simulink model "cube_3d_simulation_model_fast_mpc"  (R2016b)
settings: Solver=VariableStepAuto  StartTime=0.0  StopTime=2  RelTol=1e-3  EnableMultiTasking=on
model workspace (MAT data in the model file):
  Sig = Simulink.Signal
  Sig.DataType = 'double'
  Sig.Dimensions = -1
  Sig.DimensionsMode = 'auto'
  Sig.Complexity = 'auto'
  Sig.SampleTime = -1
  Sig.SamplingMode = 'auto'
values from neighbouring files (symbols this model uses):
  cog_offs = zeros(3,1)    [Fast_MPC_3d_Linear_system.m]    (also in Run_FastMPC_Nonlinear_model.m = theta_offs*norm(cube.rcb)*e_cog_offs)
  phi0 = deg2rad(2)    [Fast_MPC_3d_Linear_system.m]    (also in Run_FastMPC_Nonlinear_model.m = deg2rad(1.5))
  phi00 = 0    [Fast_MPC_3d_Linear_system.m]    (also in Run_FastMPC_Nonlinear_model.m)
  psi0 = deg2rad(2)    [Fast_MPC_3d_Linear_system.m]    (also in Run_FastMPC_Nonlinear_model.m = deg2rad(-1.5))
  psi00 = pi/4    (= 0.785398163397)    [Fast_MPC_3d_Linear_system.m]    (also in Run_FastMPC_Nonlinear_model.m)
  theta0 = deg2rad(2)    [Fast_MPC_3d_Linear_system.m]    (also in MPC_Parameters_3D.m = atan(sqrt(2)); Run_FastMPC_Nonlinear_model.m = deg2rad(1.5))
  theta00 = atan(sqrt(2))    [Fast_MPC_3d_Linear_system.m]    (also in Run_FastMPC_Nonlinear_model.m)
  Ts = Ts.controller    [MPC_Parameters_3D.m]
undefined symbols (not defined in the file or in its folder): cube, motor, Q0, wheel
settings Model: Creator=Love  LastModifiedBy=Wall
settings SolverCC: AlgebraicLoopSolver=LineSearch
settings OptimizationCC: LifeSpan=inf
settings DebuggingCC: SFUnexpectedBacktrackingDiag=warning  SFNoUnconditionalDefaultTransitionDiag=warning  SFExecutionAtInitializationDiag=none
settings GRTTargetCC: TargetLangStandard=C89/C90 (ANSI)  GeneratePreprocessorConditionals=Disable all
settings ConfigComp: CovMetricSettings=dw  CovHtmlReporting=on  CovSaveCumulativeToWorkspaceVar=on  CovSaveSingleToWorkspaceVar=on  CovExternalEMLEnable=off

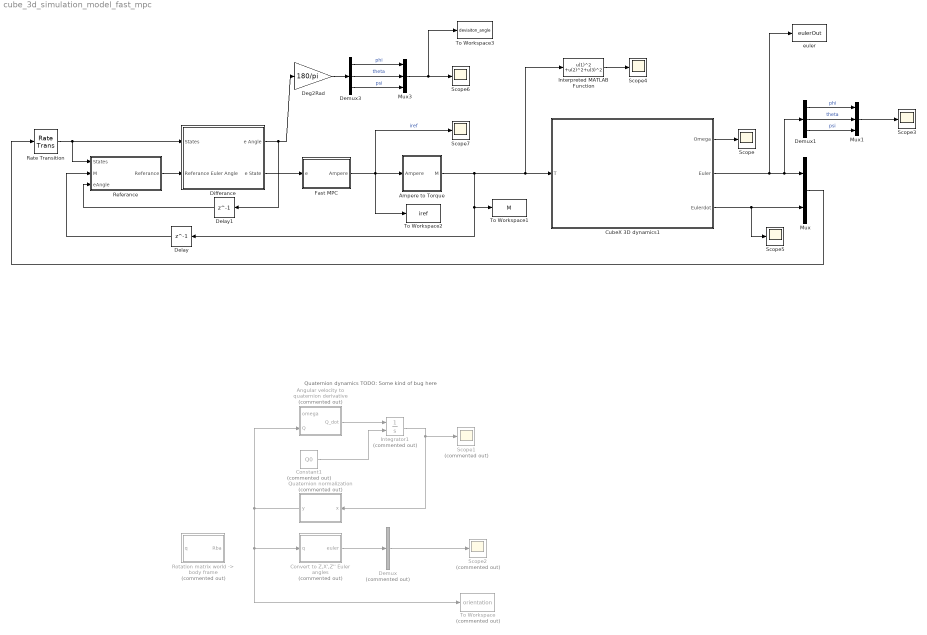
== system cube_3d_simulation_model_fast_mpc ==
  note: Quaternion dynamics TODO: Some kind of bug here
  Ampere to Torque : Subsystem
  Angular velocity to quaternion derivative : MATLAB Function  Commented=on  TreatAsAtomicUnit=on
  Constant1 : Constant  Commented=on  Value=Q0
  Convert to Z,X',Z'' Euler angles : MATLAB Function  Commented=on  TreatAsAtomicUnit=on
  CubeX 3D dynamics1 : Subsystem
  Deg2Rad : Gain  Gain=180/pi
  Delay : Delay  DelayLength=1
  Delay1 : Delay  DelayLength=1
  Demux : Demux  Commented=on  Outputs=3
  Demux1 : Demux  Outputs=3
  Demux3 : Demux  Outputs=3
  Differance : Subsystem
  Fast MPC : Subsystem
  Integrator1 : Integrator  Commented=on  InitialConditionSource=external
  Interpreted MATLAB Function : MATLABFcn  MATLABFcn=u(1)^2 +u(2)^2+u(3)^2
  Mux : Mux  Inputs=2
  Mux1 : Mux  Inputs=3
  Mux3 : Mux  Inputs=3
  Quaternion normalization : MATLAB Function  Commented=on  TreatAsAtomicUnit=on
  Rate Transition : RateTransition  OutPortSampleTime=Ts.controller
  Referance : Subsystem
  "Rotation matrix world -> body frame" : MATLAB Function  Commented=on  TreatAsAtomicUnit=on
  Scope{,3..7} (6 alike) : Scope
  Scope1 : Scope  Commented=on
  Scope2 : Scope  Commented=on
  To Workspace : ToWorkspace  Commented=on  VariableName=orientation  SaveFormat=Timeseries  SampleTime=-1
  To Workspace1 : ToWorkspace  VariableName=M  SaveFormat=Timeseries  SampleTime=-1
  To Workspace2 : ToWorkspace  VariableName=iref  SaveFormat=Timeseries  SampleTime=-1
  To Workspace3 : ToWorkspace  VariableName=deviaiton_angle  SaveFormat=Timeseries  SampleTime=-1
  "euler " : ToWorkspace  VariableName=eulerOut  SaveFormat=Timeseries  SampleTime=-1
  wires:
  Angular velocity to quaternion derivative/1(Q_dot) -> Integrator1/1
  Constant1/1 -> Integrator1/2
  Integrator1/1 -> Scope1/1, Quaternion normalization/1(x)
  Quaternion normalization/1(y) -> To Workspace/1, Convert to Z,X',Z'' Euler angles/1(q), Angular velocity to quaternion derivative/2(Q)
  Convert to Z,X',Z'' Euler angles/1(euler) -> Demux/1
  Demux/2 -> Scope2/1
  CubeX 3D dynamics1/1(Omega) -> Scope/1
  CubeX 3D dynamics1/2(Euler) -> "euler "/1, Demux1/1, Mux/1
  Mux/1 -> Rate Transition/1
  Interpreted MATLAB Function/1 -> Scope4/1
  Demux1/2 -> Mux1/2  "theta"
  Demux1/3 -> Mux1/3  "psi"
  Demux1/1 -> Mux1/1  "phi"
  Mux1/1 -> Scope3/1
  Demux3/2 -> Mux3/2  "theta"
  Demux3/3 -> Mux3/3  "psi"
  Demux3/1 -> Mux3/1  "phi"
  Deg2Rad/1 -> Demux3/1
  Mux3/1 -> To Workspace3/1, Scope6/1
  Ampere to Torque/1(M) -> To Workspace1/1, Delay/1, CubeX 3D dynamics1/1(T), Interpreted MATLAB Function/1
  Fast MPC/1(Ampere) -> To Workspace2/1, Scope7/1, Ampere to Torque/1(Ampere)  "iref"
  Rate Transition/1 -> Referance/1(States), Differance/1(States)
  Referance/1(Referance) -> Differance/2(Referance Euler Angle)
  Differance/2(e State) -> Fast MPC/1(e)
  Delay/1 -> Referance/2(M)
  Differance/1(e Angle) -> Delay1/1, Deg2Rad/1
  Delay1/1 -> Referance/3(eAngle)
  CubeX 3D dynamics1/3(Eulerdot) -> Scope5/1, Mux/2

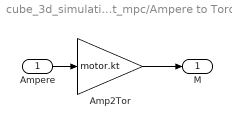
== system cube_3d_simulation_model_fast_mpc/Ampere to Torque ==
  Ampere : Inport
  Amp2Tor : Gain  Gain=motor.kt
  M : Outport
  wires:
  Amp2Tor/1 -> M/1
  Ampere/1 -> Amp2Tor/1

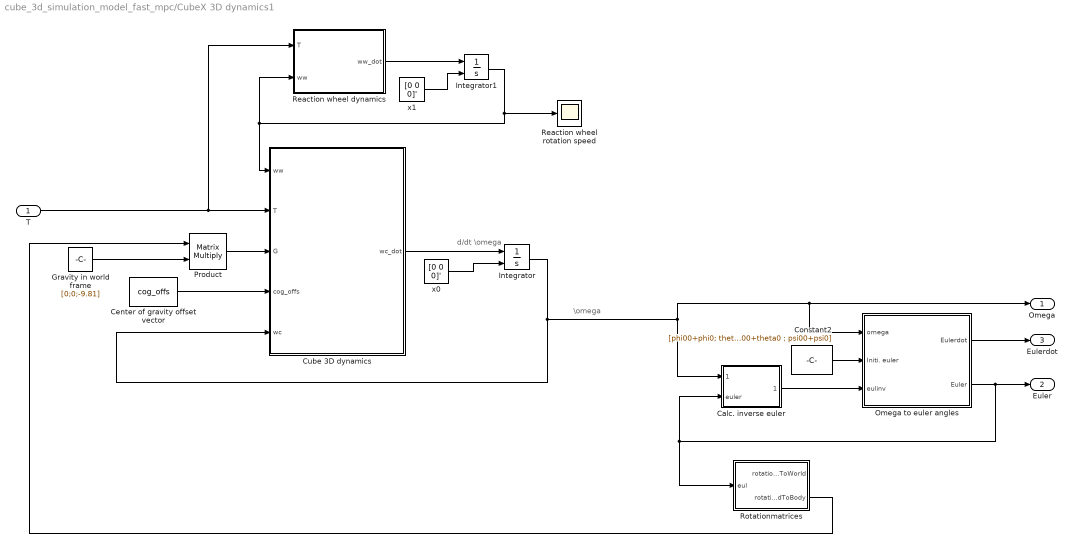
== system cube_3d_simulation_model_fast_mpc/CubeX 3D dynamics1 ==
  note: \omega
  note: d/dt \omega
  T : Inport
  Calc. inverse euler : MATLAB Function  TreatAsAtomicUnit=on
  Center of gravity offset vector : Constant  Value=cog_offs
  Constant2 : Constant  Value=[phi00+phi0; theta00+theta0 ; psi00+psi0]
  Cube 3D dynamics : MATLAB Function  TreatAsAtomicUnit=on
  Gravity in world frame : Constant  Value=[0;0;-9.81]
  Integrator : Integrator  InitialConditionSource=external
  Integrator1 : Integrator  InitialConditionSource=external
  Omega to euler angles : Subsystem
  Product : Product  Multiplication=Matrix(*)
  Reaction wheel rotation speed : Scope
  Reaction wheel dynamics : MATLAB Function  TreatAsAtomicUnit=on
  Rotationmatrices : MATLAB Function  TreatAsAtomicUnit=on
  x0 : Constant  Value=[0 0 0]'
  x1 : Constant  Value=[0 0 0]'
  Omega : Outport
  Euler : Outport  Port=2
  Eulerdot : Outport  Port=3
  wires:
  x0/1 -> Integrator/2
  Cube 3D dynamics/1(wc_dot) -> Integrator/1
  Product/1 -> Cube 3D dynamics/3(G)
  Gravity in world frame/1 -> Product/2
  Integrator/1 -> Omega/1, Omega to euler angles/1(omega), Calc. inverse euler/1(omega), Cube 3D dynamics/5(wc)
  T/1 -> Reaction wheel dynamics/1(T), Cube 3D dynamics/2(T)
  Omega to euler angles/2(Euler) -> Euler/1, Calc. inverse euler/2(euler), Rotationmatrices/1(eul)
  Constant2/1 -> Omega to euler angles/2(Initi. euler)
  Calc. inverse euler/1(EulInverse) -> Omega to euler angles/3("eulinv ")
  Rotationmatrices/2(rotationWorldToBody) -> Product/1
  Omega to euler angles/1(Eulerdot) -> Eulerdot/1
  Center of gravity offset vector/1 -> Cube 3D dynamics/4(cog_offs)
  Reaction wheel dynamics/1(ww_dot) -> Integrator1/1
  x1/1 -> Integrator1/2
  Integrator1/1 -> Reaction wheel rotation speed/1, Cube 3D dynamics/1(ww), Reaction wheel dynamics/2(ww)

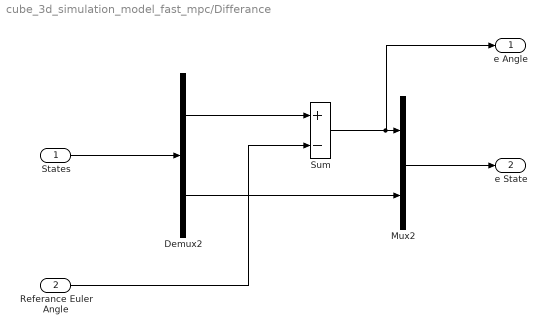
== system cube_3d_simulation_model_fast_mpc/Differance ==
  States : Inport
  Referance Euler Angle : Inport  Port=2
  Demux2 : Demux  Outputs=2
  Mux2 : Mux  Inputs=2
  Sum : Sum  Inputs=+-
  e Angle : Outport
  e State : Outport  Port=2
  wires:
  Referance Euler Angle/1 -> Sum/2
  Sum/1 -> e Angle/1, Mux2/1
  Mux2/1 -> e State/1
  Demux2/2 -> Mux2/2
  States/1 -> Demux2/1
  Demux2/1 -> Sum/1

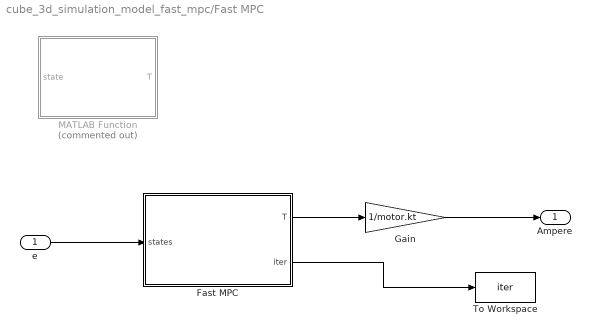
== system cube_3d_simulation_model_fast_mpc/Fast MPC ==
  e : Inport
  Fast MPC : MATLAB Function  TreatAsAtomicUnit=on
  Gain : Gain  Gain=1/motor.kt
  MATLAB Function : MATLAB Function  Commented=on  TreatAsAtomicUnit=on
  To Workspace : ToWorkspace  VariableName=iter  SaveFormat=Timeseries  SampleTime=-1
  Ampere : Outport
  wires:
  Fast MPC/1(T) -> Gain/1
  e/1 -> Fast MPC/1(states)
  Gain/1 -> Ampere/1
  Fast MPC/2(iter) -> To Workspace/1

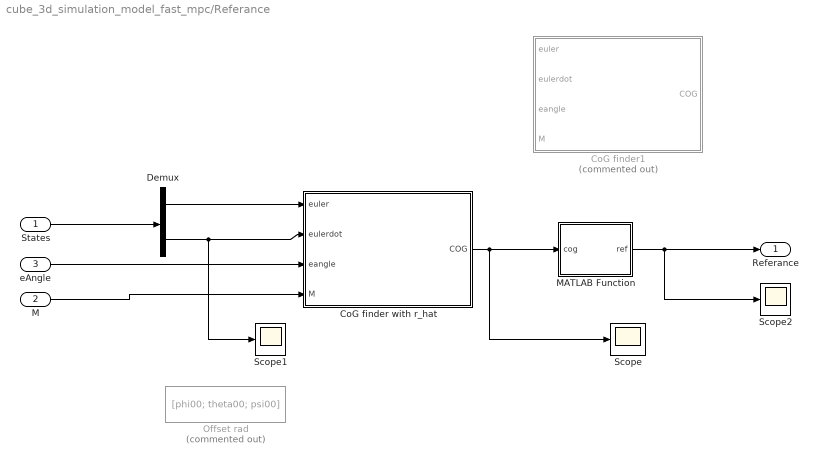
== system cube_3d_simulation_model_fast_mpc/Referance ==
  States : Inport
  M : Inport  Port=2
  eAngle : Inport  Port=3
  CoG finder with r_hat : MATLAB Function  TreatAsAtomicUnit=on
  CoG finder1 : MATLAB Function  Commented=on  TreatAsAtomicUnit=on
  Demux : Demux  Outputs=2
  MATLAB Function : MATLAB Function  TreatAsAtomicUnit=on
  Offset rad : Constant  Commented=on  Value=[phi00; theta00; psi00]  SampleTime=Ts.controller
  Scope : Scope
  Scope1 : Scope
  Scope2 : Scope
  Referance : Outport
  wires:
  MATLAB Function/1(ref) -> Referance/1, Scope2/1
  M/1 -> CoG finder with r_hat/4(M)
  States/1 -> Demux/1
  Demux/1 -> CoG finder with r_hat/1(euler)
  Demux/2 -> CoG finder with r_hat/2(eulerdot), Scope1/1
  CoG finder with r_hat/1(COG) -> MATLAB Function/1(cog), Scope/1
  eAngle/1 -> CoG finder with r_hat/3(eangle)

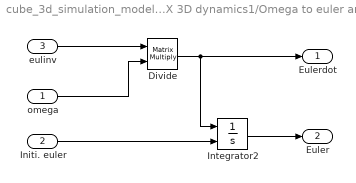
== system cube_3d_simulation_model_fast_mpc/CubeX 3D dynamics1/Omega to euler angles ==
  omega : Inport
  Initi. euler : Inport  Port=2
  "eulinv " : Inport  Port=3
  Divide : Product  Inputs=**  Multiplication=Matrix(*)
  Integrator2 : Integrator  InitialConditionSource=external
  Eulerdot : Outport
  Euler : Outport  Port=2
  wires:
  Divide/1 -> Eulerdot/1, Integrator2/1
  Initi. euler/1 -> Integrator2/2
  Integrator2/1 -> Euler/1
  omega/1 -> Divide/2
  "eulinv "/1 -> Divide/1

== matlab function cube_3d_simulation_model_fast_mpc/Angular velocity to quaternion derivative ==
  data: omega input; Q_dot output; Q input
function Q_dot = fcn(omega, Q)
%#codegen
    
   omega = omega(1:3); 
   q0=Q(1);   q1=Q(2);   q2=Q(3);   q3=Q(4);
   
   %The matrix that relates angular velocity in the body frame to the
   %quaternion derivatives. From : https://www.control.isy.liu.se/student/tsrt14/file/orientation.pdf 
   Sbar=[-q1    -q2     -q3;
          q0    -q3      q2;
          q3    q0      -q1;
         -q2    q1       q0];
    
    Q_dot = (0.5*Sbar*omega)';

== matlab function cube_3d_simulation_model_fast_mpc/CubeX 3D dynamics1/Cube 3D dynamics ==
  data: ww input; wc_dot output; T input; G input; cog_offs input; wc input; cube parameter; wheel parameter
function wc_dot = fcn(ww, T, G, cog_offs, wc, cube, wheel)
%#codegen

% T  - the torque input from the motors 
% G  - the gravity vector expressed in the body frame 
% wc - the state vector (cubes angular rate)
% ww - the reactions wheels angular rate 
% cog_offs - offset vector 
% cube - parameter struct 

%Linear momementum of the cube casing
Lc= cross(wc,(cube.I3D_tilde * wc));

% Wheel impact on the cube
Wi = cross(wc,(ww*(wheel.Iz-wheel.Iw0)));

%Gravity torque 
Tg = cross(cube.m_tot*(cube.rcb+cog_offs) + (wheel.m*wheel.rw),G);

%Eulers laws of rotation 
wdot = inv(cube.I3D)*(T + Tg - Lc + Wi);

wc_dot = wdot;

== matlab function cube_3d_simulation_model_fast_mpc/Quaternion normalization ==
  data: x input; y output
function y = fcn(x)
%#codegen

%Reportedly, numerical errors can make quaternion loose their unit length
%property. This is the remedy.  

  x(1:4)  = x(1:4) / norm(x(1:4));
  
  %Enforce q0 -> 0 to avoid ambiguity 
  if x(1) < 0,
    x(1:4) = -x(1:4);
  end

y = x;

== matlab function cube_3d_simulation_model_fast_mpc/Rotation matrix world -> body frame ==
  data: q input; Rba output
function Rba = fcn(q)
%#codegen

    R = zeros(3,3); %Added 3 dimensional result array for codegen
    
    R(1,1) = 2.*q(1).^2-1+2.*q(2).^2;
    R(1,2) = 2.*(q(2).*q(3)+q(1).*q(4));
    R(1,3) = 2.*(q(2).*q(4)-q(1).*q(3));
    R(2,1) = 2.*(q(2).*q(3)-q(1).*q(4));
    R(2,2) = 2.*q(1).^2-1+2.*q(3).^2;
    R(2,3) = 2.*(q(3).*q(4)+q(1).*q(2));
    R(3,1) = 2.*(q(2).*q(4)+q(1).*q(3));
    R(3,2) = 2.*(q(3).*q(4)-q(1).*q(2));
    R(3,3) = 2.*q(1).^2-1+2.*q(4).^2;

Rba = R';

== matlab function cube_3d_simulation_model_fast_mpc/Convert to Z,X',Z'' Euler angles ==
  data: q input; euler output
function euler = fcn(q)
%#codegen

%Convert quaternions first to parts of rotation matrix and then to Z-X'-Z''
%euler angles. Note that the angles are not the same as used in for
%instance magdwick as standard! 


    R = zeros(3,3); %Added 3 dimensional result array for codegen  
    
    R(1,3) = 2.*(q(2).*q(4)-q(1).*q(3));
     R(2,3) = 2.*(q(3).*q(4)+q(1).*q(2));
    
    R(3,1) = 2.*(q(2).*q(4)+q(1).*q(3));
    R(3,2) = 2.*(q(3).*q(4)-q(1).*q(2));
    
    R(3,3) = 2.*q(1).^2-1+2.*q(4).^2;
    
    phi = atan2(R(1,3), R(2,3)); 
    theta = acos(R(3,3)); 
    psi = atan2(  R(3,1),R(3,2) );
    
    euler = [phi;theta;psi];

== matlab function cube_3d_simulation_model_fast_mpc/CubeX 3D dynamics1/Reaction wheel dynamics ==
  data: T input; ww_dot output; ww input; wheel parameter
function ww_dot = fcn(T, ww, wheel)

% Reaction wheel dynamics

% T             - Inpu torque to the motor
% ww            - Angular rate of the wheel
% wheel.Theta_z - Inertia matrix around z axis for the wheels
% wheel.bl      - Friction coefficient.

ww_dot = inv(wheel.Theta_z) * (T - (wheel.bl*ww));

== matlab function cube_3d_simulation_model_fast_mpc/Referance/CoG finder1 ==
  data: euler input size=3; COG output size=3; eulerdot input size=3; eangle input; M input; Ts parameter; cube parameter
function COG = fcn(euler,eulerdot,eangle ,M , Ts, cube)

persistent cog L_cog

theta = euler(2);
psi = euler(3);

if isempty(cog)
   cog = zeros(3,1);
   Tf_cog = 100;         % Time Constant % 0.04
   L_cog  = Ts.controller/(Tf_cog + Ts.controller);  % Filter gain
end

if (norm(eulerdot) < .1 && norm(eulerdot) > 0  && abs(eangle(2)) < deg2rad(2) && abs(eangle(3)) < deg2rad(2) )
    mGB = -9.81 .* cube.m_tot .* [ sin(psi).*sin(theta) ; cos(psi).*sin(theta) ; cos(theta)];
    delta_r_ort =  cross(M,mGB);
    cog = (1-L_cog) * cog + L_cog * delta_r_ort;
end
COG = cog + cube.rcb;

== matlab function cube_3d_simulation_model_fast_mpc/Referance/CoG finder with r_hat ==
  data: euler input size=3; COG output size=3; eulerdot input size=3; eangle input; M input; Ts parameter; cube parameter
function COG = fcn(euler,eulerdot,eangle,M, Ts, cube)

persistent r_hat k ;

theta = euler(2);
psi = euler(3);

if isempty(r_hat)
   r_hat = zeros(3,1);
   k = 0;
end

c =  1e-5 ;

if (norm(eulerdot) < .1 && norm(eulerdot) > 0)
   
    mGB = -9.81 .* cube.m_tot .* [ sin(psi).*sin(theta) ; cos(psi).*sin(theta) ; cos(theta)];
    delta_r_ort =  cross(M,mGB);
    r_hat = r_hat + c * delta_r_ort;
end
COG = cube.rcb;

== matlab function cube_3d_simulation_model_fast_mpc/Fast MPC/Fast MPC ==
  data: states input; T output size=3; fMPC_3d parameter; iter output size=1
function [T, iter] = fcn(states, fMPC_3d)
  
    persistent lam
    
    LPD        =   double(fMPC_3d.LPD);
    LP         =   double(fMPC_3d.LP);
    D          =   double(fMPC_3d.D);
    miHDtPt    =   double(fMPC_3d.miHDtPt);
    dd         =   double(fMPC_3d.dd);
    inCo       =   double(fMPC_3d.inCo);
    nx         =   double(fMPC_3d.nx);
    N          =   double(fMPC_3d.N);
    num_of_iter=   500;
    
    if isempty(lam)
        row_of_lam = nx*N;
        assert(row_of_lam < 4096)
        lam = zeros(row_of_lam, num_of_iter);
    end
    
    w = [];


    d = dd*states;
    sig = LP * d;
    k = 2;
    while k < num_of_iter
        beta = (k-3)/k;
        mu = lam(:,k) + beta*(lam(:,k)-lam(:,k-1));
        KK = [inCo miHDtPt*mu];
        w = median(KK,2);
        lam(:,k+1) = mu + (LPD * w) - sig;

        if norm((D*w)-d,Inf) <= 1e-5
            lam(:,2) = lam(:,k);
            lam(:,3:end) = zeros(size(lam,1),num_of_iter-2);
            break;
        end
        k = k + 1;
    end
    iter = k - 1;
    T = [w(1) w(2) w(3)]';

== matlab function cube_3d_simulation_model_fast_mpc/CubeX 3D dynamics1/Calc. inverse euler ==
  data: omega input; euler input; EulInverse output
function EulInverse   = fcn(omega,euler)
%#codegen

%The relation between angular velocity in the body frame and the euler angle derivatives
%for the (Z-X',Z'') euler angle convention. 

%TODO: Get global variables to work fine
%global EulInv; 

phi     = euler(1); 
theta   = euler(2); 
psi     = euler(3); 

%Avoid the singularity at theta = 0 degrees 

theta_lim = 0.01; 
if( theta < 0 && theta > -theta_lim  )
    theta =  -theta_lim
elseif (theta > 0 && theta < theta_lim)
     theta = theta_lim; 
end

EulInverse = [csc(theta).*sin(psi),cos(psi).*csc(theta),0;cos(psi),(-1).*sin( ...
            psi),0;(-1).*cot(theta).*sin(psi),(-1).*cos(psi).*cot(theta),1];

== matlab function cube_3d_simulation_model_fast_mpc/Referance/MATLAB Function ==
  data: ref output; cog input; cube parameter
function ref = fcn(cog,cube)

rcb_tilde = cog;

rx = rcb_tilde(1); 
ry = rcb_tilde(2); 
rz = rcb_tilde(3);

psi_ref = atan2(rx, ry); 
theta_ref = atan2( sin(psi_ref)*(rx^2+ry^2),rx*rz);

ref = [0 ; theta_ref ; psi_ref ];

== matlab function cube_3d_simulation_model_fast_mpc/Fast MPC/MATLAB Function ==
  data: state input; T output size=3; MPC_3d parameter
function T = MPC(state, MPC_3d)

% Parameters

AA      =   MPC_3d.AA;             % RHS of equality constrain before multipled with state
Linv    =   MPC_3d.Linv;           % Inverse of lower-triangular Cholesky decomposition of Hessian matrix
f       =   MPC_3d.f;              % Multiplier of objective function linear term
Ain     =   MPC_3d.Ain;            % Linear inequality constraint coefficients
bin     =   MPC_3d.bin;            % Right-hand side of inequality constraints
Aeq     =   MPC_3d.Aeq;                    % Linear equality constraint coefficients
iA0     =   MPC_3d.iA0;                    % Initial active inequalities
opt     =   mpcqpsolverOptions;

beq  = AA*state;   % Right-hand side of equality constraints

[z, ~, ~, ~] =  mpcqpsolver(Linv, f', Ain, bin, Aeq, beq, iA0, opt); 

T=[z(1) z(2) z(3)]';

== matlab function cube_3d_simulation_model_fast_mpc/CubeX 3D dynamics1/Rotationmatrices ==
  data: eul input; rotationBodyToWorld output; rotationWorldToBody output
function [rotationBodyToWorld, rotationWorldToBody ] = fcn(eul)
%#codegen

%Rotation matrices from euler angles in the (Z-X'-Z'') convention 

%TODO: Get the global storage to work, seems a signal needs to be defined
%global rotationWorldToBody rotationBodyToWorld;

phi     = eul(1);
theta   = eul(2); 
psi     = eul(3); 

rotationWorldToBody= [cos(phi).*cos(psi)+(-1).*cos(theta).*sin(phi).*sin(psi),cos(psi) ...
  .*sin(phi)+cos(phi).*cos(theta).*sin(psi),sin(psi).*sin(theta);( ...
  -1).*cos(psi).*cos(theta).*sin(phi)+(-1).*cos(phi).*sin(psi),cos( ...
  phi).*cos(psi).*cos(theta)+(-1).*sin(phi).*sin(psi),cos(psi).*sin( ...
  theta);sin(phi).*sin(theta),(-1).*cos(phi).*sin(theta),cos(theta) ...
  ];

%The transpose of of orthogonal rotaation matrix gives the inverse rotation
%
rotationBodyToWorld = rotationWorldToBody';
